simulink model "simulink_continue"  (R2024b)
settings: Solver=ode45  StartTime=0.0  StopTime=1000  RelTol=1e-7  EnableMultiTasking=on
values from neighbouring files (symbols this model uses):
  gp_1 = gp_1/Gain_tec    [auto_ident_for_app.m]    (also in auto_ident_for_app_v2.m = identify(y1, u, t, 1, 0, true, NaN); auto_identification.m = gp_1 / Gain_tec)
  gp_2 = identify(y2, y1, t, 1, 0, true, 5)    [auto_ident_for_app.m]    (also in auto_ident_for_app_v2.m = identify(y2, y1, t, 1, 0, true, NaN))
  gp_3 = identify(y3, y2, t, 1, 0, false, 15)    [auto_ident_for_app.m]    (also in auto_ident_for_app_v2.m = evalin('base', 'gp_3'))
  Td = C.Kd / Kc    [actually_calculates_PID.m]
  Tf = C.Tf    [actually_calculates_PID.m]
  Ti = Kc / C.Ki    [actually_calculates_PID.m]
undefined symbols (not defined in the file or in its folder): kc, truc
settings Model: Creator=LiberT  LastModifiedBy=lordo
settings SolverCC: AlgebraicLoopSolver=TrustRegion
settings DataIOCC: LimitDataPoints=on  SaveFormat=Array  SignalLoggingSaveFormat=ModelDataLogs  ReturnWorkspaceOutputs=off
settings OptimizationCC: BlockReduction=off  BooleanDataType=off  ExpressionDepthLimit=2147483647  InitFltsAndDblsToZero=on  LifeSpan=inf
settings DebuggingCC: SaveWithParameterizedLinksMsg=none  UnderspecifiedInitializationDetection=Classic  MergeDetectMultiDrivingBlocksExec=none  SignalResolutionControl=TryResolveAllWithWarning  MultiTaskDSMMsg=warning  MultiTaskCondExecSysMsg=none  FcnCallInpInsideContextMsg=warning  UnconnectedInputMsg=warning  UnconnectedOutputMsg=warning  UnconnectedLineMsg=warning  StateNameClashWarn=warning  SFUnexpectedBacktrackingDiag=warning  SFNoUnconditionalDefaultTransitionDiag=warning  SFExecutionAtInitializationDiag=none  ArithmeticOperatorsInVariantConditions=warning
settings HardwareCC: ProdBitPerPointer=32  ProdBitPerSizeT=32  ProdBitPerPtrDiffT=32  ProdLargestAtomicFloat=None  ProdIntDivRoundTo=Undefined  ProdEndianess=Unspecified  ProdWordSize=32  ProdHWDeviceType=32-bit Generic  TargetUnknown=on
settings ModelReferenceCC: EnableRefExpFcnMdlSchedulingChecks=on  PropagateSignalLabelsOutOfModel=off
settings SFSimCC: SimUseLocalCustomCode=off  LegacyBehaviorForPersistentVarInContinuousTime=on  CustomCodeUndefinedFunction=UseInterfaceOnly
settings RTWCC: RTWUseLocalCustomCode=off  GPUComputeCapability=3.5
settings CodeAppCC: StateflowObjectComments=on
settings GRTTargetCC: TargetFcnLib=ansi_tfl_tmw.mat  TargetLangStandard=C89/C90 (ANSI)  ModelReferenceCompliant=off  CompOptLevelCompliant=off  CombineOutputUpdateFcns=off  MatFileLogging=off  GRTInterface=on
settings ConfigComp: CovMetricSettings=dw  CovSaveCumulativeToWorkspaceVar=on  CovSaveSingleToWorkspaceVar=on  CovExternalEMLEnable=off

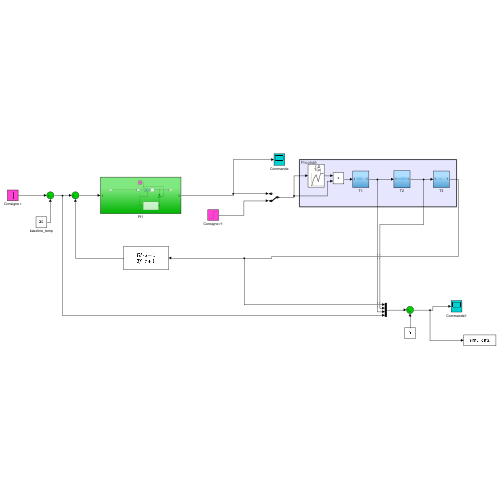
[thumbnail: Simulink's stored preview of the top-level diagram]
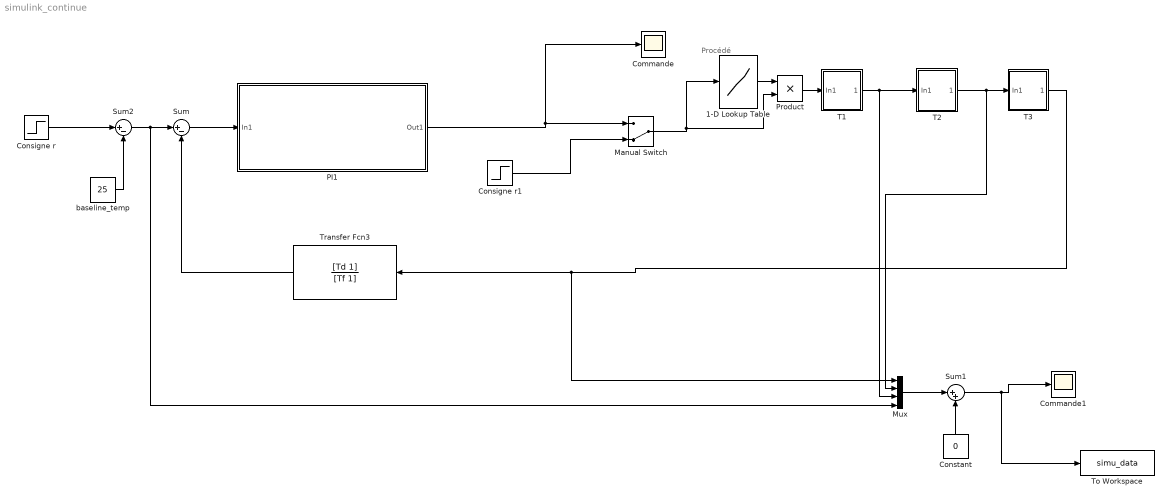
== system simulink_continue ==
  note: Procédé
  1-D Lookup Table : Lookup_n-D  NumberOfTableDimensions=1  BreakpointsForDimension1=[-0.8, -0.6, -0.4, -0.2, 0.1, 0.2, 0.4, 0.6, 0.8]  Table=[1.12, 1.62, 1.865, 2.1, 1.5, 1.72, 2.25, 2.22, 2.22]  InternalRulePriority=Speed  RndMeth=Simplest
  Commande : Scope
  Commande1 : Scope
  Consigne r : Step  Time=500  Before=30  After=20  SampleTime=0
  Consigne r1 : Step  Time=700  Before=truc{1}  After=truc{1}  SampleTime=0
  Constant : Constant  Value=0
  Manual Switch : ManualSwitch  CurrentSetting=0
  Mux : Mux
  PI1 : Subsystem
  Product : Product
  Sum : Sum  Inputs=|+-  InputSameDT=on  SaturateOnIntegerOverflow=on  OutDataTypeStr=Inherit: Same as first input
  Sum1 : Sum  Inputs=|++  InputSameDT=on  SaturateOnIntegerOverflow=on  OutDataTypeStr=Inherit: Same as first input
  Sum2 : Sum  Inputs=|+-  InputSameDT=on  SaturateOnIntegerOverflow=on  OutDataTypeStr=Inherit: Same as first input
  T1 : Subsystem
  T2 : Subsystem
  T3 : Subsystem
  To Workspace : ToWorkspace  VariableName=simu_data  SaveFormat=Structure With Time  SampleTime=-1
  Transfer Fcn3 : TransferFcn  Numerator=[Td 1]  Denominator=[Tf 1]
  baseline_temp : Constant  Value=25
  wires:
  Consigne r/1 -> Sum2/1
  baseline_temp/1 -> Sum2/2
  Sum2/1 -> Mux/4, Sum/1
  T3/1(Out1) -> Transfer Fcn3/1, Mux/1
  T2/1(Out1) -> Mux/2, T3/1(In1)
  T1/1(Out1) -> Mux/3, T2/1(In1)
  1-D Lookup Table/1 -> Product/1
  PI1/1(Out1) -> Manual Switch/1, Commande/1
  Product/1 -> T1/1(In1)
  Sum/1 -> PI1/1(In1)
  Transfer Fcn3/1 -> Sum/2
  Manual Switch/1 -> Product/2, 1-D Lookup Table/1
  Consigne r1/1 -> Manual Switch/2
  Mux/1 -> Sum1/1
  Sum1/1 -> To Workspace/1, Commande1/1
  Constant/1 -> Sum1/2

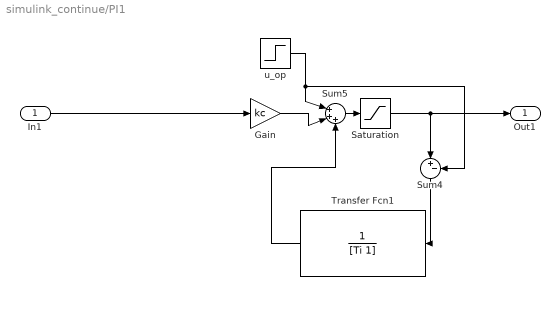
== system simulink_continue/PI1 ==
  In1 : Inport
  Gain : Gain  Gain=kc
  Saturation : Saturate  UpperLimit=1  LowerLimit=-1
  Sum4 : Sum  Inputs=|+-  InputSameDT=on  SaturateOnIntegerOverflow=on  OutDataTypeStr=Inherit: Same as first input
  Sum5 : Sum  Inputs=|+++  InputSameDT=on  SaturateOnIntegerOverflow=on  OutDataTypeStr=Inherit: Same as first input
  Transfer Fcn1 : TransferFcn  Numerator=1  Denominator=[Ti 1]
  u_op : Step  Time=0  Before=-0.00001  After=-0.00001  SampleTime=0
  Out1 : Outport
  wires:
  u_op/1 -> Sum5/1, Sum4/2
  Transfer Fcn1/1 -> Sum5/3
  Saturation/1 -> Out1/1, Sum4/1
  Sum5/1 -> Saturation/1
  Sum4/1 -> Transfer Fcn1/1
  In1/1 -> Gain/1
  Gain/1 -> Sum5/2

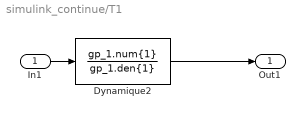
== system simulink_continue/T1 ==
  In1 : Inport
  Dynamique2 : TransferFcn  Numerator=gp_1.num{1}  Denominator=gp_1.den{1}
  Out1 : Outport
  wires:
  In1/1 -> Dynamique2/1
  Dynamique2/1 -> Out1/1

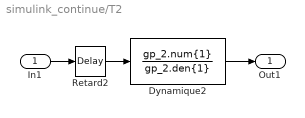
== system simulink_continue/T2 ==
  In1 : Inport
  Dynamique2 : TransferFcn  Numerator=gp_2.num{1}  Denominator=gp_2.den{1}
  Retard2 : TransportDelay  DelayTime=gp_2.IODelay  BufferSize=20000
  Out1 : Outport
  wires:
  Dynamique2/1 -> Out1/1
  In1/1 -> Retard2/1
  Retard2/1 -> Dynamique2/1

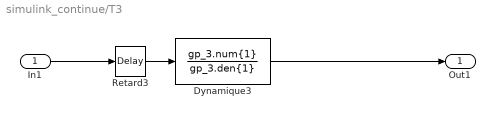
== system simulink_continue/T3 ==
  In1 : Inport
  Dynamique3 : TransferFcn  Numerator=gp_3.num{1}  Denominator=gp_3.den{1}
  Retard3 : TransportDelay  DelayTime=gp_3.IODelay  InitialOutput=0.2  BufferSize=20000
  Out1 : Outport
  wires:
  Dynamique3/1 -> Out1/1
  Retard3/1 -> Dynamique3/1
  In1/1 -> Retard3/1
